simulink model "sterowanie"  (R2018b)
settings: Solver=VariableStepAuto  StartTime=0.0  StopTime=10.0  RelTol=1e-3
undefined symbols (not defined in the file): Nieznana
libraries: simulink x1
settings Model: Creator=w-r12  LastModifiedBy=w-r12

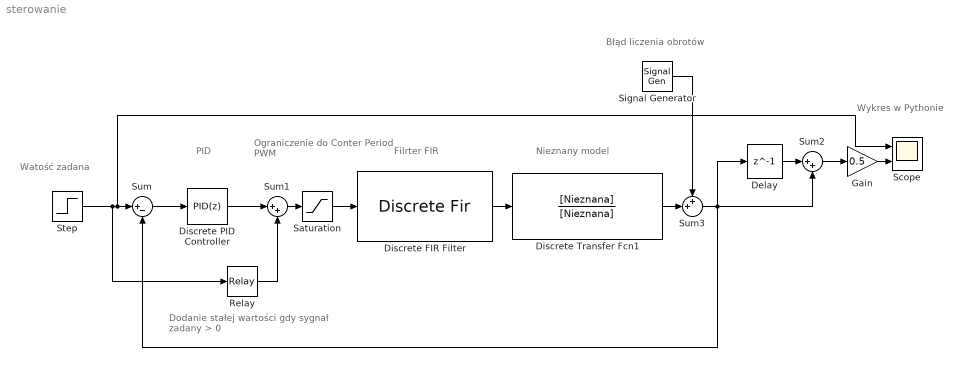
== system sterowanie ==
  note: PID
  note: Ograniczenie do
      | Conter Period PWM
  note: Filrter FIR
  note: Nieznany model
  note: Dodanie stałej wartości
      | gdy sygnał zadany > 0
  note: Watość zadana
  note: Wykres w Pythonie
  note: Błąd liczenia obrotów
  Delay : Delay  DelayLength=1  InitialCondition=0  SampleTime=0.25
  Discrete Transfer Fcn1 : DiscreteTransferFcn  Numerator=[Nieznana]  Denominator=[Nieznana]  SampleTime=0.25
  Discrete FIR Filter : DiscreteFir  Coefficients=[0.25 0.25 0.25 0.25]  InitialStates=4  SampleTime=0.25
  Discrete PID Controller : simulink/Continuous/PID Controller  Controller=PID  Form=Parallel  TimeDomain=Discrete-time  SampleTime=0.25  IntegratorMethod=Forward Euler  FilterMethod=Forward Euler  ControllerParametersSource=internal  P=1000  I=750  D=0  UseFilter=on  N=100  TunerSelectOption=Transfer Function Based (PID Tuner App)  InitialConditionSource=internal  InitialConditionForIntegrator=0  InitialConditionForFilter=0  DifferentiatorICPrevScaledInput=0  ExternalReset=none  TrackingMode=off  Kt=1  LimitOutput=off  UpperSaturationLimit=inf  LowerSaturationLimit=-inf  LinearizeAsGain=off  AntiWindupMode=none  Kb=1  POutMin=[]  POutMax=[]  IOutMin=[]  IOutMax=[]  DOutMin=[]  DOutMax=[]  NOutMin=[]  NOutMax=[]  SumOutMin=[]  SumOutMax=[]  SaturationOutMin=[]  SaturationOutMax=[]  PParamMin=[]  PParamMax=[]  IParamMin=[]  IParamMax=[]  DParamMin=[]  DParamMax=[]  NParamMin=[]  NParamMax=[]  KbParamMin=[]  KbParamMax=[]  KtParamMin=[]  KtParamMax=[]  KbOutMin=[]  KbOutMax=[]  KtOutMin=[]  KtOutMax=[]  IntegratorOutMin=[]  IntegratorOutMax=[]  FilterOutMin=[]  FilterOutMax=[]  SumI1OutMin=[]  SumI1OutMax=[]  SumI2OutMin=[]  SumI2OutMax=[]  SumI3OutMin=[]  SumI3OutMax=[]  SumI4OutMin=[]  SumI4OutMax=[]  SumDOutMin=[]  SumDOutMax=[]  DifferentiatorOutMin=[]  DifferentiatorOutMax=[]  FilterDiffOutCoefMin=[]  FilterDiffOutCoefMax=[]  ReciprocalOutMin=[]  ReciprocalOutMax=[]  SumDenOutMin=[]  SumDenOutMax=[]  SumNumOutMin=[]  SumNumOutMax=[]  DivideOutMin=[]  DivideOutMax=[]  IntegratorContinuousStateAttributes=''  IntegratorStateMustResolveToSignalObject=off  IntegratorRTWStateStorageClass=Auto  FilterContinuousStateAttributes=''  FilterStateMustResolveToSignalObject=off  FilterRTWStateStorageClass=Auto  ParallelPVariant=InternalParameters  IdealPVariant=Disabled  IVariant=InternalParameters  DVariant=InternalParameters  IntegratorVariant=Discrete  SatVariant=Disabled  AWVariant=Passthrough  PCopyVariant=Disabled  TRVariant=Disabled  FdbkBlocksVariant=Forward  IdealPFdbkVariant=Disabled  SatFdbkVariant=Disabled  DerivativeFilterVariant=ForwardEulerFilter  NVariant=InternalParameters  NCopyVariant=Disabled  FilterICVariant=InternalICsFilter  IntegratorICVariant=InternalICs  ExternalResetVariant=Disabled  TRSumVariant=Passthrough  SumFdbkVariant=Disabled  SumVariant=Sum_PID
  Gain : Gain  Gain=0.5
  Relay : Relay  OnSwitchValue=1  OffSwitchValue=0  OnOutputValue=465
  Saturation : Saturate  UpperLimit=2499  LowerLimit=0
  Scope : Scope  NumInputPorts=2
  Signal Generator : SignalGenerator  WaveForm=random  Frequency=4  VectorParams1D=off
  Step : Step  After=10  SampleTime=0
  Sum : Sum  Inputs=|+-
  Sum1 : Sum  Inputs=|++
  Sum2 : Sum  Inputs=|++
  Sum3 : Sum  Inputs=++|
  wires:
  Step/1 -> Scope/1, Sum/1, Relay/1
  Sum3/1 -> Delay/1, Sum2/2, Sum/2
  Discrete PID Controller/1 -> Sum1/1
  Sum/1 -> Discrete PID Controller/1
  Sum1/1 -> Saturation/1
  Relay/1 -> Sum1/2
  Delay/1 -> Sum2/1
  Sum2/1 -> Gain/1
  Gain/1 -> Scope/2
  Signal Generator/1 -> Sum3/1
  Discrete Transfer Fcn1/1 -> Sum3/2
  Discrete FIR Filter/1 -> Discrete Transfer Fcn1/1
  Saturation/1 -> Discrete FIR Filter/1
